simulink model "LQG"  (R2020a)
settings: Solver=VariableStepAuto  StartTime=0.0  StopTime=10  RelTol=1e-3
values from neighbouring files (symbols this model uses):
  K = lqr(sys.A,sys.B,Q,R)    [LQGControl.m]    (also in LQRControl.m; LQRcontrol_with_Integrator.m; MPC.m = 0.028)
  NL = 1    [LQGControl.m]    (also in LQRControl.m = 0)
  Rn = 10    [Blocks_LQR.m]    (also in Blocks_LQRbasic.m = 0.01; LQGControl.m = 0.0001; LQRControl.m = 0.0001; LQRcontrol_with_Integrator.m)
  sys = ss(A,B,C,D)    [Blocks_LQR.m]    (also in Blocks_LQRbasic.m; MPC.m = ss(a,b,c,d))
  ts = 0.01    [LQGControl.m]    (also in LQRControl.m; LQRcontrol_with_Integrator.m)
  x0 = zeros(12,1)    [Blocks_LQR.m]    (also in LQGControl.m; LQRControl.m; LQRcontrol_with_Integrator.m; animation_LQG.m = 10)
undefined symbols (not defined in the file or in its folder): Continuous, Time
libraries: simulink x10, ctrlSharedLib x1
settings Model: Creator=blaze8871  LastModifiedBy=blaze8871
settings DataIOCC: SaveTime=off

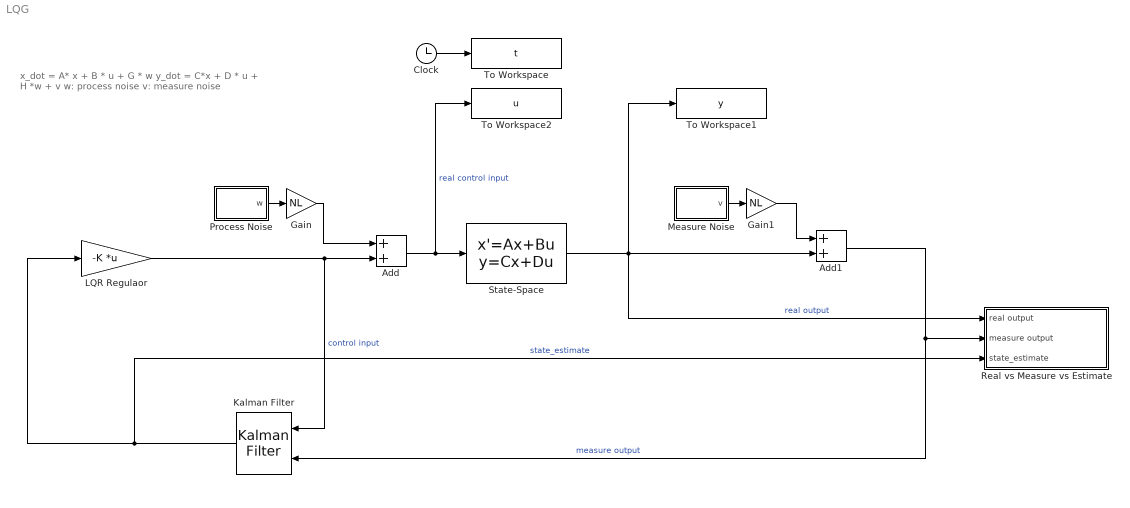
== system LQG ==
  note: x_dot = A* x + B * u + G * w
      | y_dot = C*x + D * u + H *w + v
      |
      | w: process noise
      | v: measure noise
  Add : Sum
  Add1 : Sum
  Clock : Clock
  Gain : Gain  Gain=NL
  Gain1 : Gain  Gain=NL
  Kalman Filter : ctrlSharedLib/Kalman Filter  TimeDomain=Continuous-Time  UseCurrentEstimator=on  ModelSource=Individual A, B, C, D matrices  ModelSourceVariable=ss(0.95,1,1,0,1)  A=sys.A  B=sys.B  C=sys.C  D=sys.D  NumberOfStates=1  NumberOfInputs=1  NumberOfOutputs=1  InitialEstimateSource=Dialog  X0=x0  P0=10  UseK=off  UseGH=off  NumberOfProcessNoiseInputs=1  G=G  TimeInvariantG=on  H=0  TimeInvariantH=on  Q=Qn  TimeInvariantQ=on  R=Rn  TimeInvariantR=on  N=0  TimeInvariantN=on  AddInputPort=on  AddEnablePort=off  OutputEstimatedY=off  OutputP=off  Ts=-1
  LQR Regulaor : Gain  Gain=-K  Multiplication=Matrix(K*u)
  Measure Noise : Subsystem
  Process Noise : Subsystem
  Real vs Measure vs Estimate : Subsystem
  State-Space : StateSpace  A=sys.A  B=sys.B  C=sys.C  D=sys.D  InitialCondition=x0
  To Workspace : ToWorkspace  VariableName=t  SampleTime=0.01
  To Workspace1 : ToWorkspace  VariableName=y  SampleTime=0.01
  To Workspace2 : ToWorkspace  VariableName=u  SampleTime=0.01
  wires:
  State-Space/1 -> Add1/2, Real vs Measure vs Estimate/1(real output), To Workspace1/1  "real output"
  Add1/1 -> Real vs Measure vs Estimate/2(measure output), Kalman Filter/2  "measure output"
  Clock/1 -> To Workspace/1
  Add/1 -> State-Space/1, To Workspace2/1  "real control input"
  Kalman Filter/1 -> Real vs Measure vs Estimate/3(state_estimate), LQR Regulaor/1  "state_estimate"
  LQR Regulaor/1 -> Kalman Filter/1, Add/2  "control input"
  Process Noise/1(w) -> Gain/1
  Measure Noise/1(v) -> Gain1/1
  Gain/1 -> Add/1
  Gain1/1 -> Add1/1

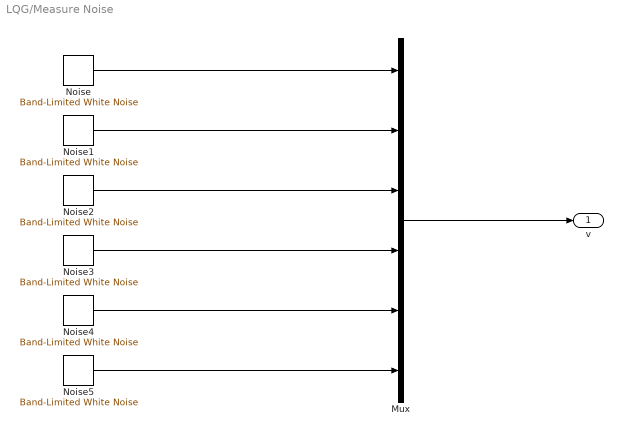
== system LQG/Measure Noise ==
  " Noise" : simulink/Sources/Band-Limited White Noise  Cov=Rn*ts  Ts=ts  seed=[11432]
  " Noise1" : simulink/Sources/Band-Limited White Noise  Cov=Rn*ts  Ts=ts  seed=[13242]
  " Noise2" : simulink/Sources/Band-Limited White Noise  Cov=Rn*ts  Ts=ts  seed=[34124]
  " Noise3" : simulink/Sources/Band-Limited White Noise  Cov=Rn*ts  Ts=ts  seed=[41123]
  " Noise4" : simulink/Sources/Band-Limited White Noise  Cov=Rn*ts  Ts=ts  seed=[32144]
  " Noise5" : simulink/Sources/Band-Limited White Noise  Cov=Rn*ts  Ts=ts  seed=[14123]
  Mux : Mux  Inputs=6
  v : Outport
  wires:
  Mux/1 -> v/1
  " Noise3"/1 -> Mux/4
  " Noise2"/1 -> Mux/3
  " Noise1"/1 -> Mux/2
  " Noise"/1 -> Mux/1
  " Noise4"/1 -> Mux/5
  " Noise5"/1 -> Mux/6

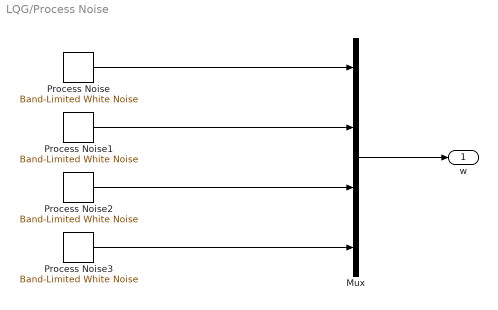
== system LQG/Process Noise ==
  Mux : Mux
  Process Noise : simulink/Sources/Band-Limited White Noise  Cov=1e-3*ts  Ts=ts  seed=[11432]
  Process Noise1 : simulink/Sources/Band-Limited White Noise  Cov=1e-3*ts  Ts=ts  seed=[13242]
  Process Noise2 : simulink/Sources/Band-Limited White Noise  Cov=1e-3*ts  Ts=ts  seed=[34124]
  Process Noise3 : simulink/Sources/Band-Limited White Noise  Cov=1e-3*ts  Ts=ts  seed=[41123]
  w : Outport
  wires:
  Process Noise/1 -> Mux/1
  Mux/1 -> w/1
  Process Noise1/1 -> Mux/2
  Process Noise2/1 -> Mux/3
  Process Noise3/1 -> Mux/4

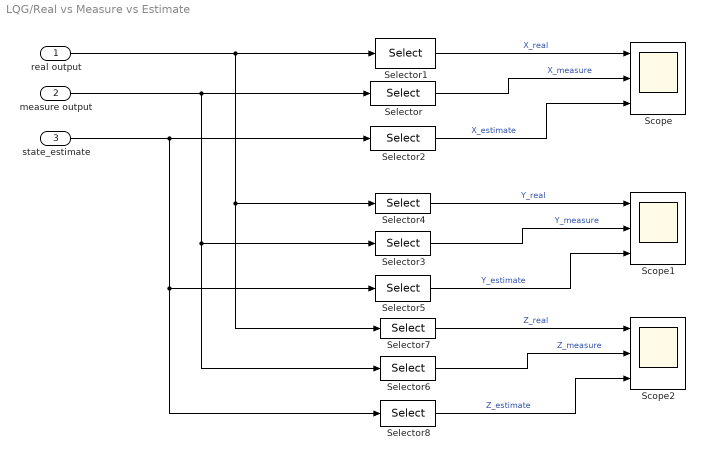
== system LQG/Real vs Measure vs Estimate ==
  real output : Inport
  measure output : Inport  Port=2
  state_estimate : Inport  Port=3
  Scope : Scope  NumInputPorts=3
  Scope1 : Scope  NumInputPorts=3
  Scope2 : Scope  NumInputPorts=3
  Selector : Selector  InputPortWidth=6  IndexOptions=Index vector (dialog)  Indices=[1]  OutputSizes=1
  Selector1 : Selector  InputPortWidth=6  IndexOptions=Index vector (dialog)  Indices=[1]  OutputSizes=1
  Selector2 : Selector  InputPortWidth=12  IndexOptions=Index vector (dialog)  Indices=[4]  OutputSizes=1
  Selector3 : Selector  InputPortWidth=6  IndexOptions=Index vector (dialog)  Indices=[2]  OutputSizes=1
  Selector4 : Selector  InputPortWidth=6  IndexOptions=Index vector (dialog)  Indices=[2]  OutputSizes=1
  Selector5 : Selector  InputPortWidth=12  IndexOptions=Index vector (dialog)  Indices=[5]  OutputSizes=1
  Selector6 : Selector  InputPortWidth=6  IndexOptions=Index vector (dialog)  Indices=[3]  OutputSizes=1
  Selector7 : Selector  InputPortWidth=6  IndexOptions=Index vector (dialog)  Indices=[3]  OutputSizes=1
  Selector8 : Selector  InputPortWidth=12  IndexOptions=Index vector (dialog)  Indices=[6]  OutputSizes=1
  wires:
  Selector2/1 -> Scope/3  "X_estimate"
  Selector1/1 -> Scope/1  "X_real"
  Selector/1 -> Scope/2  "X_measure"
  Selector3/1 -> Scope1/2  "Y_measure"
  Selector4/1 -> Scope1/1  "Y_real"
  Selector5/1 -> Scope1/3  "Y_estimate"
  real output/1 -> Selector4/1, Selector7/1, Selector1/1
  Selector8/1 -> Scope2/3  "Z_estimate"
  Selector7/1 -> Scope2/1  "Z_real"
  Selector6/1 -> Scope2/2  "Z_measure"
  measure output/1 -> Selector6/1, Selector3/1, Selector/1
  state_estimate/1 -> Selector8/1, Selector5/1, Selector2/1
